simulink subsystem "Subsystem_Controlador"  (R2023b)
settings: Solver=VariableStepAuto  StartTime=0.0  StopTime=10.0  RelTol=1e-3
libraries: arduinolib x2
settings Model: Creator=Alberto  LastModifiedBy=Alberto

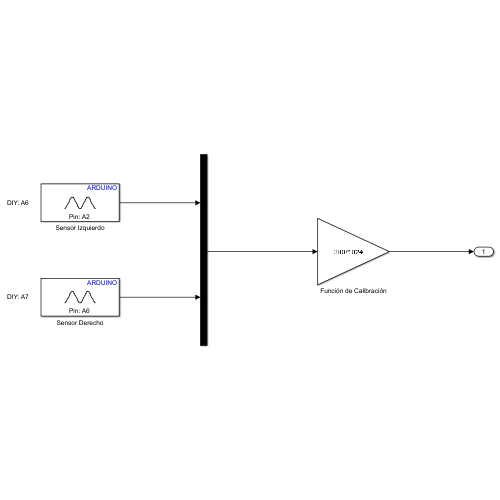
[thumbnail: Simulink's stored preview of the top-level diagram]
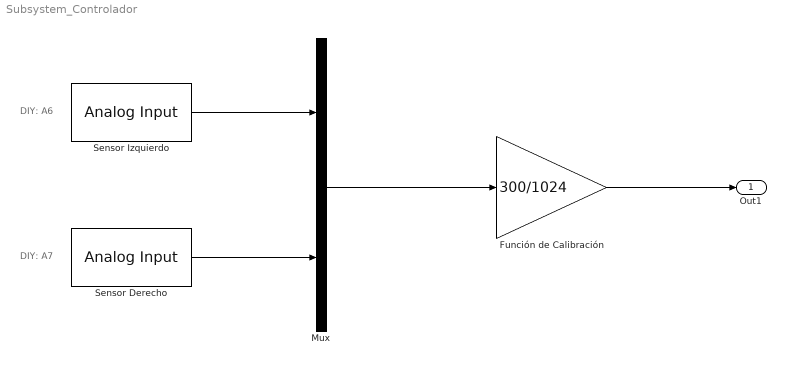
== system Subsystem_Controlador ==
  note: DIY: A7
  note: DIY: A6
  Función de Calibración : Gain  Gain=300/1024
  Mux : Mux  Inputs=2
  Sensor Derecho : arduinolib/Analog Input  pinNumber=6  ReadResultsOnly=off  ConversionTriggerSource=Software  ExternalTriggerType=uint32( 0 )  OutputDataType=uint16  EnableConversionCompleteNotify=off  EnableOuputStatus=off  SampleTime=-1  blockPlatform=arduino
  Sensor Izquierdo : arduinolib/Analog Input  pinNumber=2  ReadResultsOnly=off  ConversionTriggerSource=Software  ExternalTriggerType=uint32( 0 )  OutputDataType=uint16  EnableConversionCompleteNotify=off  EnableOuputStatus=off  SampleTime=-1  blockPlatform=arduino
  Out1 : Outport
  wires:
  Función de Calibración/1 -> Out1/1
  Sensor Derecho/1 -> Mux/2
  Sensor Izquierdo/1 -> Mux/1
  Mux/1 -> Función de Calibración/1
